simulink model "model_sample"  (R2019b)
settings: Solver=FixedStepDiscrete  StartTime=0.0  StopTime=10.0  RelTol=1e-3  EnableMultiTasking=on
settings Model: SimulationMode=external  Creator=guest  LastModifiedBy=gurtnmar
settings DataIOCC: ReturnWorkspaceOutputs=off
settings OptimizationCC: PassReuseOutputArgsAs=Individual arguments  EfficientTunableParamExpr=on
settings DebuggingCC: ParameterTunabilityLossMsg=error  ArithmeticOperatorsInVariantConditions=warning
settings SFSimCC: SimUseLocalCustomCode=off  MATLABDynamicMemAlloc=off  CustomCodeUndefinedFunction=UseInterfaceOnly
settings RTWCC: Description=Linux Embedded Coder  SystemTargetFile=ert_linux.tlc  MakeCommand="make_rtw OPT_OPTS=\"-O2 -ggdb -Wall\" CC=aarch64-linux-gnu-gcc CPP=aarch64-linux-gnu-gcc"  TemplateMakefile=ert_linux.tmf  GenerateReport=on  RTWUseLocalCustomCode=off  IncludeHyperlinkInReport=on  LaunchReport=on  GenerateTraceInfo=on  GenerateTraceReport=on  GenerateTraceReportSl=on  GenerateTraceReportSf=on  GenerateTraceReportEml=on
settings CodeAppCC: ForceParamTrailComments=on  IgnoreCustomStorageClasses=off  OperatorAnnotations=on  SimulinkDataObjDesc=on  SFDataObjDesc=on  MATLABFcnDesc=on  InsertBlockDesc=on  StateflowObjectComments=on  MATLABSourceComments=on
settings STFCustomTargetCC: TargetLangStandard=C99 (ISO)  MultiwordLength=256  ModelReferenceCompliant=off  CombineOutputUpdateFcns=on  ERTCustomFileBanners=on  SupportContinuousTime=off  RemoveResetFunc=on  MATLABClassNameForMDSCustomization=Simulink.SoftwareTarget.ERTCustomization  SystemTargetFile=ert_linux.tlc
settings ERTTargetCC: TargetLangStandard=C99 (ISO)  ModelReferenceCompliant=off  ParMdlRefBuildCompliant=off  CompOptLevelCompliant=off  ConcurrentExecutionCompliant=off  SupportNonInlinedSFcns=on  ModelStepFunctionPrototypeControlCompliant=off  CPPClassGenCompliant=off  UseToolchainInfoCompliant=off  ExtMode=on  ExtModeMexArgs='147.32.86.138'  ERTCustomFileTemplate=ert_linux_file_process.tlc

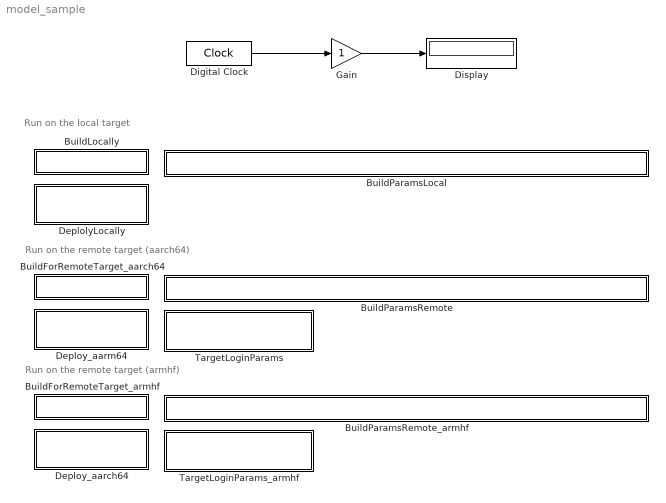
== system model_sample ==
  note: Run on the remote target (armhf)
  note: Run on the local target
  note: Run on the remote target (aarch64)
  BuildForRemoteTarget_aarch64 : Subsystem
      settings: OpenFcn=ert_linux_build(gcs, 'BuildParamsRemote');
      mask Display: disp('Build')
  BuildForRemoteTarget_armhf : Subsystem
      settings: OpenFcn=ert_linux_build(gcs, 'BuildParamsRemote_armhf')
      mask Display: disp('Build')
  BuildLocally : Subsystem
      settings: OpenFcn=ert_linux_build(gcs, 'BuildParamsLocal');
      mask Display: disp('Build')
  BuildParamsLocal : Subsystem  mask{make_command='make_rtw OPT_OPTS="-O2 -ggdb -Wall" CC=gcc'}
      mask prompts: make_command "MakeCommand"
      mask Display: disp(get_param(gcb, 'make_command'));
  BuildParamsRemote : Subsystem  mask{make_command='make_rtw OPT_OPTS="-O2 -ggdb -Wall" CC=aarch64-linux-gnu-gcc CPP=aarch64-linux-gnu-gcc'}
      mask prompts: make_command "MakeCommand"
      mask Display: disp(get_param(gcb, 'make_command'));
  BuildParamsRemote_armhf : Subsystem  mask{make_command='make_rtw OPT_OPTS="-O2 -ggdb -Wall" CC=arm-linux-gnueabihf-gcc CPP=arm-linux-gnueabihf-gcc'}
      mask prompts: make_command "MakeCommand"
      mask Display: disp(get_param(gcb, 'make_command'));
  DeplolyLocally : Subsystem
      settings: OpenFcn=ert_linux_deploy_and_connect(gcs);
      mask Display: disp('Deploy and\nconnect')
  Deploy_aarch64 : Subsystem
      settings: OpenFcn=ert_linux_deploy_and_connect(gcs, 'TargetLoginParams_armhf');
      mask Display: disp('Deploy and\nconnect')
  Deploy_aarm64 : Subsystem
      settings: OpenFcn=ert_linux_deploy_and_connect(gcs, 'TargetLoginParams');
      mask Display: disp('Deploy and\nconnect')
  Digital Clock : DigitalClock
  Display : Display
  Gain : Gain
  TargetLoginParams : Subsystem  mask{trgt_ip_addr='192.168.1.5', trgt_username='user'}
      mask prompts: trgt_ip_addr "Target IP address"; trgt_username "Target username"
      mask Display:
      | ip_addr = get_param(gcb, 'trgt_ip_addr');
      | user = get_param(gcb, 'trgt_username');
      | 
      | fprintf('IP addr:\t %s\n User:\t %s ', ip_addr, user);
  TargetLoginParams_armhf : Subsystem  mask{trgt_ip_addr='192.168.1.10', trgt_username='user'}
      mask prompts: trgt_ip_addr "Target IP address"; trgt_username "Target username"
      mask Display:
      | ip_addr = get_param(gcb, 'trgt_ip_addr');
      | user = get_param(gcb, 'trgt_username');
      | 
      | fprintf('IP addr:\t %s\n User:\t %s ', ip_addr, user);
  wires:
  Digital Clock/1 -> Gain/1
  Gain/1 -> Display/1

== system model_sample/BuildForRemoteTarget_aarch64 ==

== system model_sample/BuildForRemoteTarget_armhf ==

== system model_sample/BuildLocally ==

== system model_sample/BuildParamsLocal ==

== system model_sample/BuildParamsRemote ==

== system model_sample/BuildParamsRemote_armhf ==

== system model_sample/DeplolyLocally ==

== system model_sample/Deploy_aarch64 ==

== system model_sample/Deploy_aarm64 ==

== system model_sample/TargetLoginParams ==

== system model_sample/TargetLoginParams_armhf ==
